simulink model "sampleModel1940_sub"  (R2023a)
settings: Solver=VariableStepAuto  StartTime=0.0  StopTime=10.0  RelTol=1e-3
libraries: hdlsllib x6, simulink x1
settings Model: Creator=user1  LastModifiedBy=user1

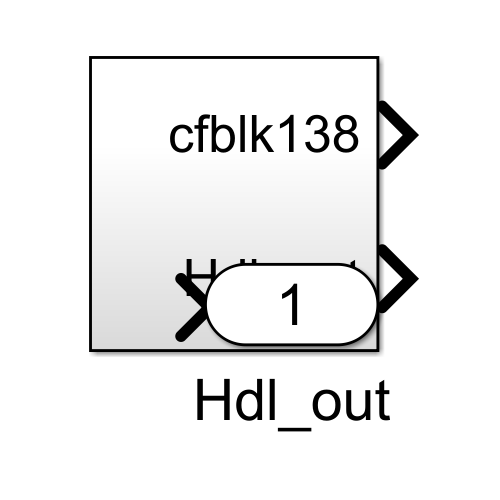
[thumbnail: Simulink's stored preview of the top-level diagram]
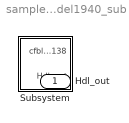
== system sampleModel1940_sub ==
  Subsystem : Subsystem
  Hdl_out : Outport  OutDataTypeStr=uint8

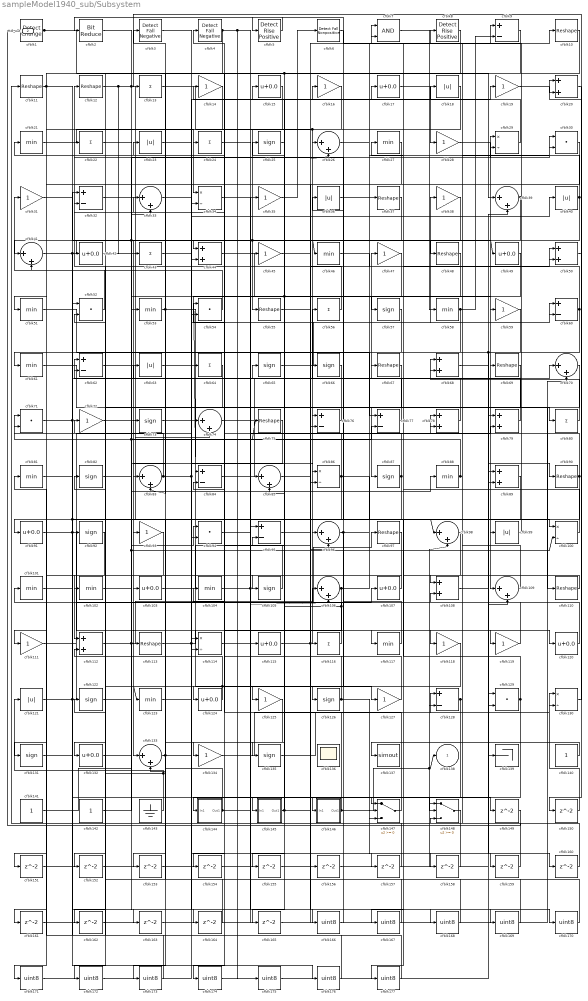
== system sampleModel1940_sub/Subsystem ==
  cfblk1 : simulink/Logic and Bit Operations/Detect Change  vinit=0  OutDataTypeStr=uint8
      settings: LibrarySourceBlock=|
      | hdlsllib/Logic and Bit
      | Operations/Detect
      | Change
  cfblk{10..12,37,48,55,67,69,75,90,97,110,113} (13 alike) : Reshape
  cfblk{29,34,86,100,114,130} (6 alike) : Product  Inputs=*/  OutDataTypeStr=uint8  RndMeth=Zero  SaturateOnIntegerOverflow=on
  cfblk{21,27,46,51,53,58,61,81,88,101..102,104,117,123} (14 alike) : MinMax  OutDataTypeStr=uint8
  cfblk{15,17,42,49,91,103,107,115,120,124,132} (11 alike) : Bias  Bias=0.0  SaturateOnIntegerOverflow=off
  cfblk{25,57,65..66,73,82,87,92,105,122,126,131,135} (13 alike) : Signum
  cfblk{26,33,39,41,70,74,83,85,96,98,106,109,133} (13 alike) : Sum  Inputs=|++  OutDataTypeStr=uint8
  cfblk{20,44,50,68,78..79,89,108,112} (9 alike) : Sum  OutDataTypeStr=uint8
  cfblk{14,16,19,28,31,35,38,45,47,59,72,93,111,118..119,125,127,134} (18 alike) : Gain  OutDataTypeStr=uint8
  cfblk{13,22,24,43,56,64,80,116} (8 alike) : Sum  Inputs=+  OutDataTypeStr=uint8
  cfblk{18,23,36,40,63,99,121} (7 alike) : Abs  OutDataTypeStr=uint8  SaturateOnIntegerOverflow=off
  cfblk{9,32,60,62,76..77,84,95,128} (9 alike) : Sum  Inputs=+-  OutDataTypeStr=uint8
  cfblk{30,52,54,71,94,129} (6 alike) : DotProduct  OutDataTypeStr=uint8
  cfblk136 : Scope
      settings: Floating=on
  cfblk137 : ToWorkspace  VariableName=simout  SaveFormat=Timeseries  SampleTime=-1
  cfblk139 : Terminator
  cfblk140 : Constant  OutDataTypeStr=uint8  SampleTime=-1
  cfblk141 : Constant  OutDataTypeStr=uint8  SampleTime=-1
  cfblk142 : Constant  OutDataTypeStr=uint8  SampleTime=-1
  cfblk143 : Ground
  cfblk144 : Subsystem
      settings: LibrarySourceBlock=|
      | hdlsllib/Ports &
      | Subsystems/Subsystem
  cfblk145 : Subsystem
      settings: LibrarySourceBlock=|
      | hdlsllib/Ports &
      | Subsystems/Subsystem
  cfblk146 : Subsystem
      settings: LibrarySourceBlock=|
      | hdlsllib/Ports &
      | Subsystems/Subsystem
  cfblk147 : Switch  OutDataTypeStr=uint8  SaturateOnIntegerOverflow=off  InputSameDT=off
  cfblk148 : Switch  OutDataTypeStr=uint8  SaturateOnIntegerOverflow=off  InputSameDT=off
  cfblk{149..165} (17 alike) : Delay  SampleTime=1
  cfblk{166..177} (12 alike) : DataTypeConversion  OutDataTypeStr=uint8  SaturateOnIntegerOverflow=off  RndMeth=Floor
  cfblk2 : hdlsllib/Logic and Bit Operations/Bit Reduce  mode=AND
  cfblk3 : hdlsllib/Logic and Bit Operations/Detect Fall Negative  vinit=0  OutDataTypeStr=uint8
  cfblk4 : hdlsllib/Logic and Bit Operations/Detect Fall Negative  vinit=0  OutDataTypeStr=uint8
  cfblk5 : hdlsllib/Logic and Bit Operations/Detect Rise Positive  vinit=0  OutDataTypeStr=uint8
  cfblk6 : hdlsllib/Logic and Bit Operations/Detect Fall Nonpositive  vinit=0  OutDataTypeStr=uint8
  cfblk7 : Logic  AllPortsSameDT=off  OutDataTypeStr=boolean
  cfblk8 : hdlsllib/Logic and Bit Operations/Detect Rise Positive  vinit=0  OutDataTypeStr=uint8
  cfblk138 : Outport  OutDataTypeStr=uint8  VectorParamsAs1DForOutWhenUnconnected=off
  Hdl_out : Outport  Port=2  OutDataTypeStr=uint8
  wires:
  cfblk70/1 -> cfblk133/1
  cfblk16/1 -> cfblk34/2, cfblk116/1
  cfblk15/1 -> cfblk55/1
  cfblk63/1 -> cfblk127/1
  cfblk28/1 -> cfblk109/1
  cfblk35/1 -> cfblk6/1
  cfblk120/1 -> cfblk101/1
  cfblk110/1 -> cfblk108/1
  cfblk147/1 -> cfblk15/1
  cfblk14/1 -> cfblk34/1
  cfblk132/1 -> cfblk100/2, cfblk94/1
  cfblk48/1 -> cfblk105/1
  cfblk12/1 -> cfblk43/1, cfblk86/2, cfblk86/1
  cfblk38/1 -> cfblk103/1
  cfblk112/1 -> cfblk77/2, cfblk97/1
  cfblk57/1 -> cfblk134/1
  cfblk96/1 -> cfblk10/1, cfblk126/1
  cfblk79/1 -> cfblk62/1
  cfblk76/1 -> cfblk56/1
  cfblk56/1 -> cfblk12/1
  cfblk47/1 -> cfblk165/1, cfblk84/1
  cfblk9/1 -> cfblk155/1, cfblk154/1
  cfblk78/1 -> cfblk47/1
  cfblk65/1 -> cfblk38/1
  cfblk119/1 -> cfblk108/2
  cfblk113/1 -> cfblk40/1, cfblk119/1
  cfblk146/1(Out1) -> cfblk54/1, cfblk98/2, cfblk138/1
  cfblk21/1 -> cfblk24/1
  cfblk115/1 -> cfblk26/2, cfblk148/2
  cfblk33/1 -> cfblk19/1
  cfblk105/1 -> cfblk4/1
  cfblk39/1 -> cfblk83/1, cfblk5/1
  cfblk102/1 -> cfblk53/1
  cfblk52/1 -> cfblk31/1
  cfblk134/1 -> cfblk130/1
  cfblk121/1 -> cfblk147/2, cfblk107/1
  cfblk72/1 -> cfblk100/1
  cfblk61/1 -> cfblk139/1
  cfblk83/1 -> cfblk71/2, cfblk147/3, cfblk60/1
  cfblk87/1 -> cfblk91/1, cfblk25/1
  cfblk50/1 -> cfblk13/1
  cfblk80/1 -> cfblk68/1
  cfblk94/1 -> cfblk35/1
  cfblk130/1 -> cfblk20/1
  cfblk90/1 -> cfblk147/1, cfblk32/2
  cfblk117/1 -> cfblk22/1
  cfblk18/1 -> cfblk41/1
  cfblk7/1 -> cfblk58/1
  cfblk1/1 -> Hdl_out/1, cfblk39/1
  cfblk140/1 -> cfblk137/1
  cfblk19/1 -> cfblk20/2
  cfblk64/1 -> cfblk132/1
  cfblk106/1 -> cfblk174/1, cfblk30/1
  cfblk100/1 -> cfblk27/1
  cfblk69/1 -> cfblk93/1
  cfblk11/1 -> cfblk51/1, cfblk44/1
  cfblk84/1 -> cfblk67/1
  cfblk40/1 -> cfblk18/1, cfblk124/1
  cfblk75/1 -> cfblk94/2
  cfblk91/1 -> cfblk113/1
  cfblk99/1 -> cfblk29/1
  cfblk71/1 -> cfblk65/1, cfblk146/1(In1), cfblk98/1
  cfblk25/1 -> cfblk145/1(In1)
  cfblk60/1 -> cfblk7/2, cfblk61/1
  cfblk32/1 -> cfblk115/1
  cfblk126/1 -> cfblk158/1, cfblk84/2
  cfblk53/1 -> cfblk83/2, cfblk110/1
  cfblk34/1 -> cfblk118/1
  cfblk44/1 -> cfblk69/1
  cfblk73/1 -> cfblk76/1
  cfblk77/1 -> cfblk33/1
  cfblk111/1 -> cfblk60/2
  cfblk93/1 -> cfblk112/1
  cfblk6/1 -> cfblk96/1
  cfblk148/1 -> cfblk11/1
  cfblk107/1 -> cfblk102/1
  cfblk74/1 -> cfblk80/1
  cfblk67/1 -> cfblk87/1
  cfblk68/1 -> cfblk90/1
  cfblk109/1 -> cfblk16/1
  cfblk143/1 -> cfblk122/1, cfblk121/1
  cfblk131/1 -> cfblk66/1
  cfblk85/1 -> cfblk70/1
  cfblk129/1 -> cfblk177/1, cfblk17/1
  cfblk86/1 -> cfblk21/1, cfblk111/1, cfblk99/1
  cfblk144/1(Out1) -> cfblk79/2, cfblk23/1
  cfblk142/1 -> cfblk33/2
  cfblk133/1 -> cfblk63/1, cfblk64/1
  cfblk31/1 -> cfblk45/1, cfblk49/1
  cfblk13/1 -> cfblk26/1
  cfblk135/1 -> cfblk128/1
  cfblk62/1 -> cfblk74/2
  cfblk51/1 -> cfblk77/1
  cfblk4/1 -> cfblk162/1, cfblk175/1, cfblk117/1
  cfblk103/1 -> cfblk50/1
  cfblk123/1 -> cfblk30/2
  cfblk10/1 -> cfblk73/1
  cfblk22/1 -> cfblk120/1, cfblk46/1
  cfblk124/1 -> cfblk42/1, cfblk123/1
  cfblk116/1 -> cfblk85/2, cfblk106/1
  cfblk128/1 -> cfblk78/2, cfblk144/1(In1)
  cfblk46/1 -> cfblk50/2
  cfblk58/1 -> cfblk9/2, cfblk125/1
  cfblk41/1 -> cfblk48/1, cfblk164/1, cfblk92/1
  cfblk24/1 -> cfblk95/1
  cfblk2/1 -> cfblk59/1
  cfblk141/1 -> cfblk75/1, cfblk29/2
  cfblk55/1 -> cfblk7/1
  cfblk5/1 -> cfblk2/1
  cfblk36/1 -> cfblk37/1
  cfblk145/1(Out1) -> cfblk159/1, cfblk95/2
  cfblk88/1 -> cfblk71/1, cfblk8/1
  cfblk127/1 -> cfblk104/1
  cfblk66/1 -> cfblk62/2
  cfblk17/1 -> cfblk28/1
  cfblk42/1 -> cfblk54/2
  cfblk26/1 -> cfblk9/1
  cfblk8/1 -> cfblk131/1
  cfblk30/1 -> cfblk76/2
  cfblk104/1 -> cfblk78/1, cfblk106/2
  cfblk29/1 -> cfblk14/1
  cfblk49/1 -> cfblk57/1
  cfblk59/1 -> cfblk129/2, cfblk135/1
  cfblk122/1 -> cfblk88/1
  cfblk54/1 -> cfblk41/2
  cfblk23/1 -> cfblk149/1
  cfblk149/1 -> cfblk1/1
  cfblk20/1 -> cfblk150/1
  cfblk150/1 -> cfblk130/2
  cfblk27/1 -> cfblk151/1
  cfblk151/1 -> cfblk74/1
  cfblk118/1 -> cfblk152/1
  cfblk152/1 -> cfblk109/2
  cfblk125/1 -> cfblk153/1
  cfblk153/1 -> cfblk79/1
  cfblk154/1 -> cfblk148/1
  cfblk155/1 -> cfblk128/2
  cfblk95/1 -> cfblk156/1
  cfblk156/1 -> cfblk39/2
  cfblk43/1 -> cfblk157/1
  cfblk157/1 -> cfblk32/1
  cfblk158/1 -> cfblk148/3
  cfblk159/1 -> cfblk133/2
  cfblk108/1 -> cfblk160/1
  cfblk160/1 -> cfblk68/2
  cfblk92/1 -> cfblk161/1
  cfblk161/1 -> cfblk44/2
  cfblk162/1 -> cfblk96/2
  cfblk101/1 -> cfblk163/1
  cfblk163/1 -> cfblk85/1
  cfblk164/1 -> cfblk112/2
  cfblk165/1 -> cfblk70/2
  cfblk3/1 -> cfblk166/1
  cfblk166/1 -> cfblk36/1
  cfblk98/1 -> cfblk167/1
  cfblk167/1 -> cfblk3/1
  cfblk82/1 -> cfblk168/1
  cfblk168/1 -> cfblk72/1
  cfblk45/1 -> cfblk169/1
  cfblk169/1 -> cfblk82/1
  cfblk114/1 -> cfblk170/1
  cfblk170/1 -> cfblk129/1
  cfblk37/1 -> cfblk171/1
  cfblk171/1 -> cfblk114/1
  cfblk97/1 -> cfblk172/1
  cfblk172/1 -> cfblk114/2
  cfblk89/1 -> cfblk173/1
  cfblk173/1 -> cfblk52/2
  cfblk174/1 -> cfblk89/1
  cfblk175/1 -> cfblk89/2
  cfblk81/1 -> cfblk176/1
  cfblk176/1 -> cfblk52/1
  cfblk177/1 -> cfblk81/1

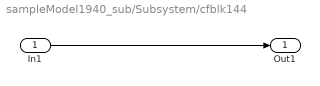
== system sampleModel1940_sub/Subsystem/cfblk144 ==
  In1 : Inport
  Out1 : Outport
  wires:
  In1/1 -> Out1/1

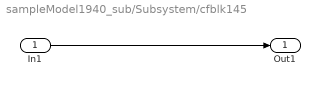
== system sampleModel1940_sub/Subsystem/cfblk145 ==
  In1 : Inport
  Out1 : Outport
  wires:
  In1/1 -> Out1/1

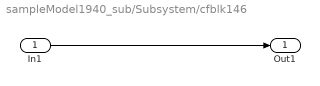
== system sampleModel1940_sub/Subsystem/cfblk146 ==
  In1 : Inport
  Out1 : Outport
  wires:
  In1/1 -> Out1/1
